simulink model "ChargeMgmt"  (R2022b)
settings: configuration reference "BMS_Sw_CodeGenConfig" (kept outside this file)
values from neighbouring files (symbols this model uses):
  currentFactor = 20.0    [DD_ChargeMgmt.sldd]
  CV_Gain = 0.5    [DD_ChargeMgmt.sldd]
  MaxCellVoltThrsld = 4.15    [DD_ChargeMgmt.sldd]
  MaxChrgCurrLim = 3.3    [DD_CurrPowerLimCalc.sldd]
  noCurrent = 0.0    [DD_ChargeMgmt.sldd]
  voltThreshold = 4.1    [DD_ChargeMgmt.sldd]
undefined symbols (not defined in the file or in its folder): Np_Module
settings Model: DataDictionary=DD_ChargeMgmt.sldd  Creator=cpatel  LastModifiedBy=cpatel
settings ConfigSetRef: SourceName=BMS_Sw_CodeGenConfig

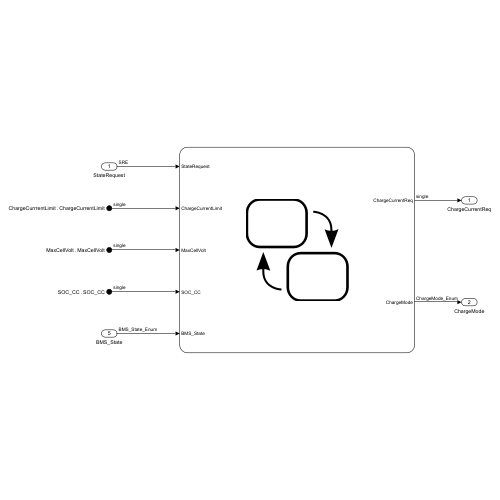
[thumbnail: Simulink's stored preview of the top-level diagram]
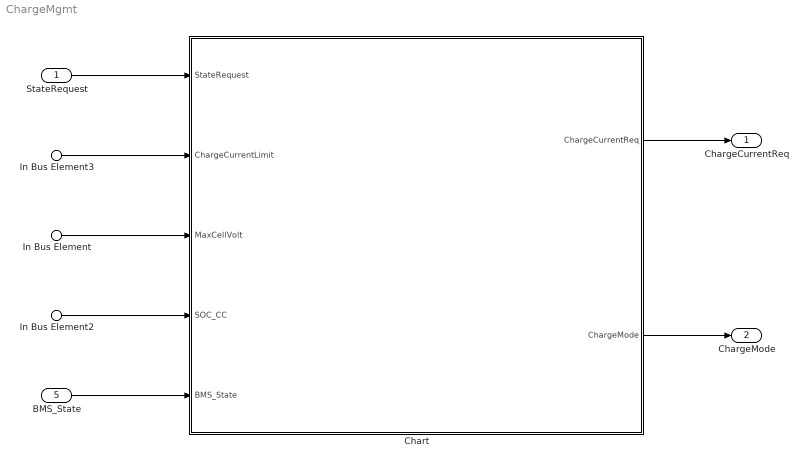
== system ChargeMgmt ==
  StateRequest : Inport  OutDataTypeStr=Enum: SRE
  In Bus Element3 : Inport  Port=2  PortName=ChargeCurrrentLimit  Element=ChargeCurrentLimit
  In Bus Element : Inport  Port=3  PortName=MaxCellVolt  Element=MaxCellVolt
  In Bus Element2 : Inport  Port=4  PortName=SOC_CC  Element=SOC_CC
  BMS_State : Inport  Port=5  OutDataTypeStr=Enum: BMS_State_Enum
  Chart : Stateflow chart  TreatAsAtomicUnit=on
  ChargeCurrentReq : Outport
  ChargeMode : Outport  Port=2
  wires:
  In Bus Element3/1 -> Chart/2(ChargeCurrentLimit)
  In Bus Element/1 -> Chart/3(MaxCellVolt)
  In Bus Element2/1 -> Chart/4(SOC_CC)
  Chart/1(ChargeCurrentReq) -> ChargeCurrentReq/1
  StateRequest/1 -> Chart/1(StateRequest)
  Chart/2(ChargeMode) -> ChargeMode/1
  BMS_State/1 -> Chart/5(BMS_State)

== stateflow chart ChargeMgmt/Chart ==
  state ChrgStandby
    en:
    ChargeMode = ChargeMode_Enum.ChrgStandby;
    ChargeCurrentReq = noCurrent;
  state ChrgCC
    en:
    ChargeMode = ChargeMode_Enum.CC;
    du:
    ChargeCurrentReq = ChargeCurrentLimit;
  state ChrgCV
    en:
    ChargeMode = ChargeMode_Enum.CV;
    du:
    ChargeCurrentReq = ChargeCurrentReq - CV_Gain*(MaxCellVolt - MaxCellVoltThrsld);
    ChargeCurrentReq = min(ChargeCurrentReq, ChargeCurrentLimit);
  (default) -> ChrgStandby
  ChrgCV -> ChrgStandby : [StateRequest ~= SRE.Charging || ...
      | ChargeCurrentReq <= (MaxChrgCurrLim*Np_Module/currentFactor) || ...
      | max(SOC_CC) >single(0.98)]
  ChrgCC -> ChrgStandby [order 1] : [StateRequest ~= SRE.Charging]
  ChrgStandby -> ChrgCC : [StateRequest == SRE.Charging && ...
      | BMS_State == BMS_State_Enum.BMS_Charging && ...
      | MaxCellVolt < voltThreshold && ...
      | max(SOC_CC) < single(0.95)]
  ChrgCC -> ChrgCV [order 2] : [MaxCellVolt>=...
      | MaxCellVoltThrsld]
  data: StateRequest input; ChargeCurrentLimit input; MaxCellVolt input; SOC_CC input; ChargeCurrentReq output; CV_Gain parameter; voltThreshold parameter; noCurrent parameter; MaxCellVoltThrsld parameter; Np_Module parameter; currentFactor parameter; MaxChrgCurrLim parameter; ChargeMode output; BMS_State input
